simulink library "MBDyn_collision_activator"  (R2016b)
settings: Solver=VariableStepAuto  StartTime=0.0  StopTime=10.0  RelTol=1e-3
values from neighbouring files (symbols this model uses):
  coefficient_viscous_friction = 0.05    [multiple_points_platform_and_ball_characteristics.m]
  restitution_coefficient = 0.2    [multiple_points_platform_and_ball_characteristics.m]
undefined symbols (not defined in the file or in its folder): dz_at_rest, platform_damping_factor
undefined symbols (not defined in the file): Coulomb_friction_value, ctflag_threshold, delta_z_rest, dz_threshold, mu_z
libraries: simulink x4
settings Model: Creator=matteo  LastModifiedBy=matteo

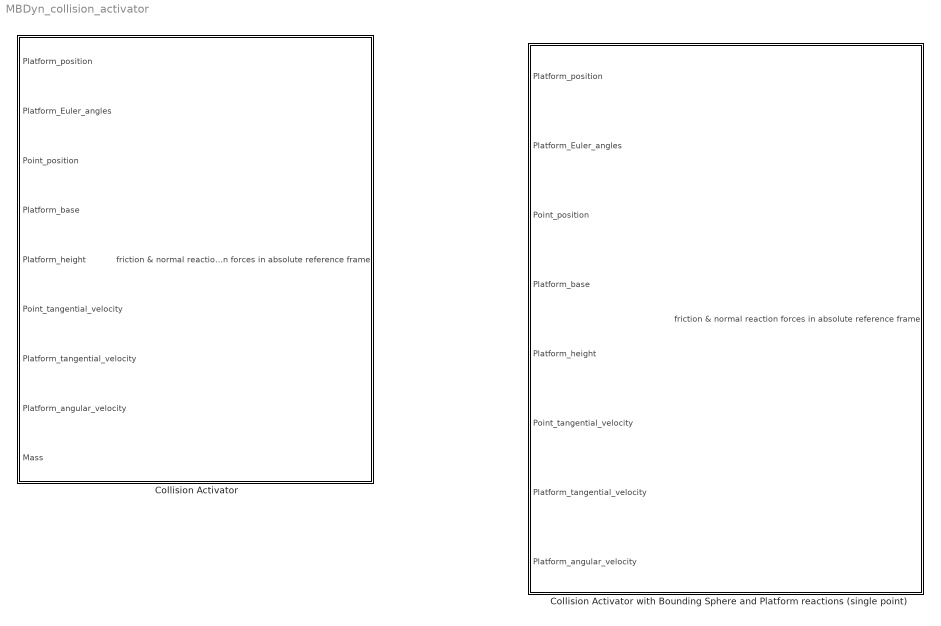
== system MBDyn_collision_activator ==
  Collision Activator : Subsystem  mask{coulomb_friction_value=Coulomb_friction_value, coefficient_viscous_friction=coefficient_viscous_friction, cosine_flag_threshold=ctflag_threshold, local_distance_from_gnd_threshold=dz_threshold, platform_damping_factor=mu_z, dz_at_rest=delta_z_rest}
      mask prompts: coulomb_friction_value "Coulomb friction value (offset)"; coefficient_viscous_friction "coefficient of viscous friction (gain)"; cosine_flag_threshold "cosine flag threshold"; local_distance_from_gnd_threshold "local distance from ground threshold"; platform_damping_factor "platform damping factor"; dz_at_rest "desired_platform deformation at rest"
      mask DialogControl MBDyn_collision_activator Prompt: MBDyn collision activator. Author: Matteo Daniele. This block models a simple point-to-rectangular platform collision interaction.
  Collision Activator with Bounding Sphere and Platform reactions (single point) : Subsystem  mask{mult_factor=10, coulomb_friction_value=0, coefficient_viscous_friction=0.05, cosine_flag_threshold=3.9, local_distance_from_gnd_threshold=0, ground_stiffness=1e9, restitution_coeff=0.8, impact_speed_threshold=0.2, reaction_force_exponential=3, force_sign=-1, dissipation_coefficient_model=Flores}
      mask prompts: mult_factor "bounding sphere platform multiplication factor"; coulomb_friction_value "Coulomb friction value (offset)"; coefficient_viscous_friction "coefficient of viscous friction (gain)"; cosine_flag_threshold "cosine flag threshold"; local_distance_from_gnd_threshold "local distance from ground threshold"; ground_stiffness "normal reaction stiffness"; restitution_coeff "restitution coefficient"; impact_speed_threshold "impact speed threshold"; reaction_force_exponential "reaction force exponential"; force_sign "reaction force sign (+1 or -1)"; dissipation_coefficient_model "dissipation coefficient model"
      mask TypeOptions dissipation_coefficient_model: Flores | Hunt Crossley | Lankarani Nikravesh
      mask DialogControl MBDyn_collision_activator Prompt: MBDyn collision activator. Author: Matteo Daniele. This block models a simple point-to-rectangular platform collision interaction.

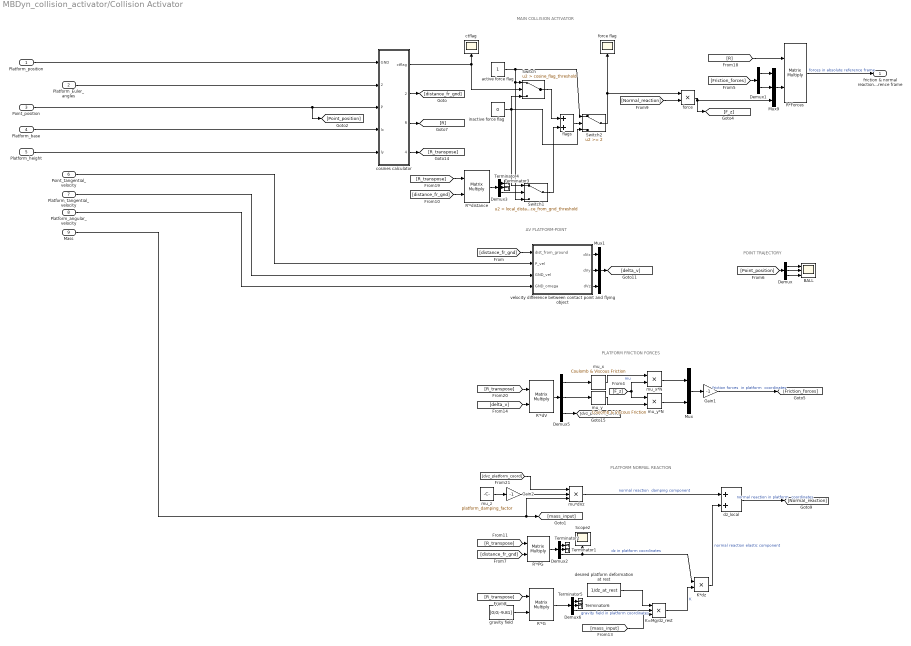
== system MBDyn_collision_activator/Collision Activator ==
  note: PLATFORM NORMAL REACTION
  note: PLATFORM FRICTION FORCES
  note: POINT TRAJECTORY
  note: ΔV PLATFORM-POINT
  note: MAIN COLLISION ACTIVATOR
  Platform_position : Inport
  Platform_Euler_angles : Inport  Port=2
  Point_position : Inport  Port=3
  Platform_base : Inport  Port=4
  Platform_height : Inport  Port=5
  Point_tangential_velocity : Inport  Port=6
  Platform_tangential_velocity : Inport  Port=7
  Platform_angular_velocity : Inport  Port=8
  Mass : Inport  Port=9
  BALL : Scope  NumInputPorts=3
  Demux{,2..3,5..6} (5 alike) : Demux  Outputs=3
  Demux1 : Demux  Outputs=2
  Gain1 : Gain  Gain=-1
  Gain2 : Gain  Gain=-1
  K*dz : Product
  K=Mg/dz_rest : Product  Inputs=3
  Mux : Mux  Inputs=2
  Mux1 : Mux  Inputs=3
  Mux9 : Mux  Inputs=3
  R'*G : Product  Multiplication=Matrix(*)
  R'*PG : Product  Multiplication=Matrix(*)
  R'*dV : Product  Multiplication=Matrix(*)
  R'*distance : Product  Multiplication=Matrix(*)
  R*Forces : Product  Multiplication=Matrix(*)
  Scope2 : Scope
  Switch : Switch  Criteria=u2 > Threshold  Threshold=cosine_flag_threshold
  Switch1 : Switch  Criteria=u2 > Threshold  Threshold=local_distance_from_gnd_threshold
  Switch2 : Switch  Threshold=2
  Terminator{1..6} (6 alike) : Terminator
  active force flag : Constant
  cosines calculator : MATLAB Function  TreatAsAtomicUnit=on
  ctflag : Scope
  desired platform deformation at rest : Constant  Value=1/dz_at_rest
  dz_local : Sum
  flags : Sum
  force : Product
  force flag : Scope
  gravity field : Constant  Value=[0;0;-9.81]
  inactive force flag : Constant  Value=0
  mu*dVz : Product  Inputs=3
  mu_x : simulink/Discontinuities/Coulomb & Viscous Friction  offset=coulomb_friction_value  gain=coefficient_viscous_friction
  mu_x*N : Product
  mu_y : simulink/Discontinuities/Coulomb & Viscous Friction  offset=coulomb_friction_value  gain=coefficient_viscous_friction
  mu_y*N : Product
  mu_z : Constant  Value=platform_damping_factor
  velocity difference between contact point and flying object : MATLAB Function  TreatAsAtomicUnit=on
  friction & normal reaction forces in absolute reference frame : Outport
  wires:
  active force flag/1 -> Switch/1, Switch1/3, Switch2/1
  dz_local/1 -> [Normal_reaction]  "normal reaction in platform  coordinates"
  Platform_height/1 -> cosines calculator/5(ly)
  cosines calculator/3(R) -> [R]
  cosines calculator/2(distance_PG) -> [distance_fr_gnd]
  [mass_input] -> K=Mg/dz_rest/3
  Demux6/3 -> K=Mg/dz_rest/2  "gravity field in platform coordinates"
  Platform_position/1 -> cosines calculator/1(GND)
  mu_y*N/1 -> Mux/2
  Demux5/3 -> [dvz_platform_coord]
  Demux2/2 -> Terminator1/1
  K=Mg/dz_rest/1 -> K*dz/2  "K"
  velocity difference between contact point and flying object/2(dVy) -> Mux1/2
  [distance_fr_gnd] -> R'*PG/2
  Demux/3 -> BALL/3
  [distance_fr_gnd] -> R'*distance/2
  Demux2/1 -> Terminator2/1
  Point_tangential_velocity/1 -> velocity difference between contact point and flying object/2(P_vel)
  Gain1/1 -> [Friction_forces]  "friction forces  in platform  coordinates"
  R*Forces/1 -> friction & normal reaction forces in absolute reference frame/1  "forces in absolute reference frame"
  Demux/1 -> BALL/1
  inactive force flag/1 -> Switch/3, Switch1/1, Switch2/3
  mu_x*N/1 -> Mux/1
  Platform_Euler_angles/1 -> cosines calculator/2(GND_Phi)
  Demux3/2 -> Terminator3/1
  mu*dVz/1 -> dz_local/1  "normal reaction  damping component"
  [F_z] -> mu_y*N/1, mu_x*N/2
  cosines calculator/1(ctflag) -> Switch/2, ctflag/1
  mu_y/1 -> mu_y*N/2
  Platform_tangential_velocity/1 -> velocity difference between contact point and flying object/3(GND_vel)
  Mux9/1 -> R*Forces/2
  velocity difference between contact point and flying object/1(dVx) -> Mux1/1
  [R_transpose] -> R'*G/1
  [R_transpose] -> R'*distance/1
  R'*dV/1 -> Demux5/1
  Point_position/1 -> cosines calculator/3(P), [Point_position]
  Gain2/1 -> mu*dVz/2
  R'*PG/1 -> Demux2/1
  Mass/1 -> mu*dVz/3, [mass_input]
  [Normal_reaction] -> force/2
  mu_x/1 -> mu_x*N/1  "mu"
  Mux1/1 -> [delta_v]
  [Point_position] -> Demux/1
  Switch2/1 -> force/1, force flag/1
  Demux1/2 -> Mux9/2
  Platform_angular_velocity/1 -> velocity difference between contact point and flying object/4(GND_omega)
  [R_transpose] -> R'*PG/1
  Demux6/1 -> Terminator5/1
  Demux3/3 -> Switch1/2
  Demux1/1 -> Mux9/1
  [R_transpose] -> R'*dV/1
  [Friction_forces] -> Demux1/1
  K*dz/1 -> dz_local/2  "normal reaction elastic component"
  Switch/1 -> flags/1
  force/1 -> [F_z], Mux9/3
  Demux/2 -> BALL/2
  Demux6/2 -> Terminator6/1
  flags/1 -> Switch2/2
  desired platform deformation at rest/1 -> K=Mg/dz_rest/1
  [distance_fr_gnd] -> velocity difference between contact point and flying object/1(dist_from_ground)
  Mux/1 -> Gain1/1
  mu_z/1 -> Gain2/1
  Demux3/1 -> Terminator4/1
  [dvz_platform_coord] -> mu*dVz/1
  cosines calculator/4(R_global_to_local) -> [R_transpose]
  Demux5/1 -> mu_x/1
  Demux5/2 -> mu_y/1
  velocity difference between contact point and flying object/3(dVz) -> Mux1/3
  R'*distance/1 -> Demux3/1
  R'*G/1 -> Demux6/1
  [R] -> R*Forces/1
  gravity field/1 -> R'*G/2
  [delta_v] -> R'*dV/2
  Switch1/1 -> flags/2
  Platform_base/1 -> cosines calculator/4(lx)
  Demux2/3 -> Scope2/1, K*dz/1  "dz in platform coordinates"

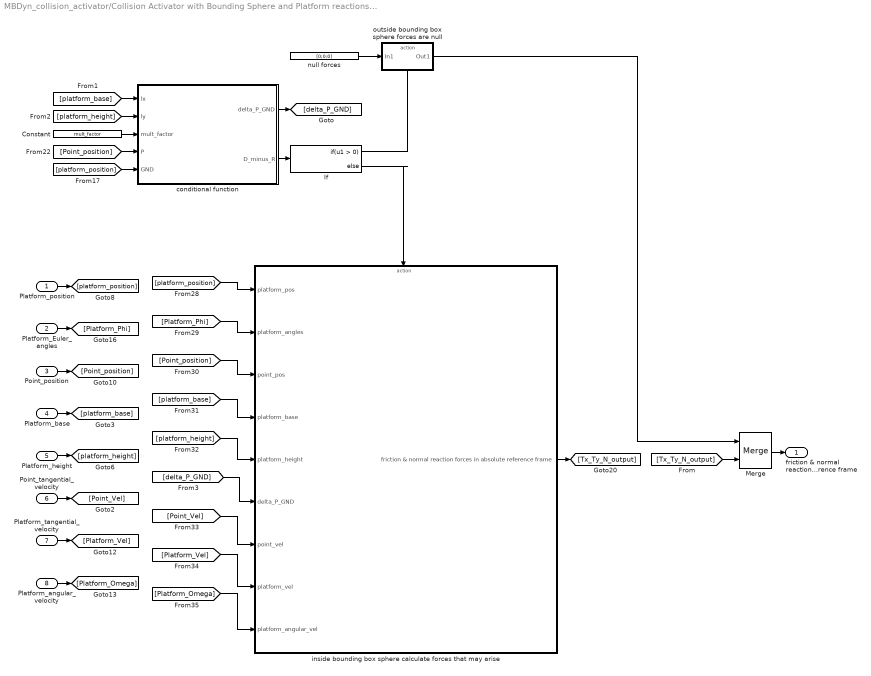
== system MBDyn_collision_activator/Collision Activator with Bounding Sphere and Platform reactions (single point) ==
  Platform_position : Inport
  Platform_Euler_angles : Inport  Port=2
  Point_position : Inport  Port=3
  Platform_base : Inport  Port=4
  Platform_height : Inport  Port=5
  Point_tangential_velocity : Inport  Port=6
  Platform_tangential_velocity : Inport  Port=7
  Platform_angular_velocity : Inport  Port=8
  Constant : Constant  Value=mult_factor
  If : If
  Merge : Merge
  conditional function : MATLAB Function  TreatAsAtomicUnit=on
  inside bounding box sphere calculate forces that may arise : Subsystem  TreatAsAtomicUnit=on
  null forces : Constant  Value=[0;0;0]
  outside bounding box sphere forces are null : Subsystem  TreatAsAtomicUnit=on
  friction & normal reaction forces in absolute reference frame : Outport
  wires:
  [delta_P_GND] -> inside bounding box sphere calculate forces that may arise/6(delta_P_GND)
  inside bounding box sphere calculate forces that may arise/1(friction & normal reaction forces in absolute reference frame) -> [Tx_Ty_N_output]
  null forces/1 -> outside bounding box sphere forces are null/1(In1)
  If/1 -> outside bounding box sphere forces are null/Action
  If/2 -> inside bounding box sphere calculate forces that may arise/Action
  [Platform_Omega] -> inside bounding box sphere calculate forces that may arise/9(platform_angular_vel)
  [Platform_Vel] -> inside bounding box sphere calculate forces that may arise/8(platform_vel)
  [Point_Vel] -> inside bounding box sphere calculate forces that may arise/7(point_vel)
  [platform_height] -> inside bounding box sphere calculate forces that may arise/5(platform_height)
  [platform_base] -> inside bounding box sphere calculate forces that may arise/4(platform_base)
  [Point_position] -> inside bounding box sphere calculate forces that may arise/3(point_pos)
  [Platform_Phi] -> inside bounding box sphere calculate forces that may arise/2(platform_angles)
  [platform_position] -> inside bounding box sphere calculate forces that may arise/1(platform_pos)
  conditional function/2(D_minus_R) -> If/1
  conditional function/1(delta_P_GND) -> [delta_P_GND]
  [Tx_Ty_N_output] -> Merge/2
  outside bounding box sphere forces are null/1(Out1) -> Merge/1
  Merge/1 -> friction & normal reaction forces in absolute reference frame/1
  Platform_Euler_angles/1 -> [Platform_Phi]
  Point_tangential_velocity/1 -> [Point_Vel]
  Platform_tangential_velocity/1 -> [Platform_Vel]
  Platform_angular_velocity/1 -> [Platform_Omega]
  [Point_position] -> conditional function/4(P)
  [platform_position] -> conditional function/5(GND)
  Constant/1 -> conditional function/3(mult_factor)
  Point_position/1 -> [Point_position]
  Platform_position/1 -> [platform_position]
  [platform_height] -> conditional function/2(ly)
  [platform_base] -> conditional function/1(lx)
  Platform_height/1 -> [platform_height]
  Platform_base/1 -> [platform_base]

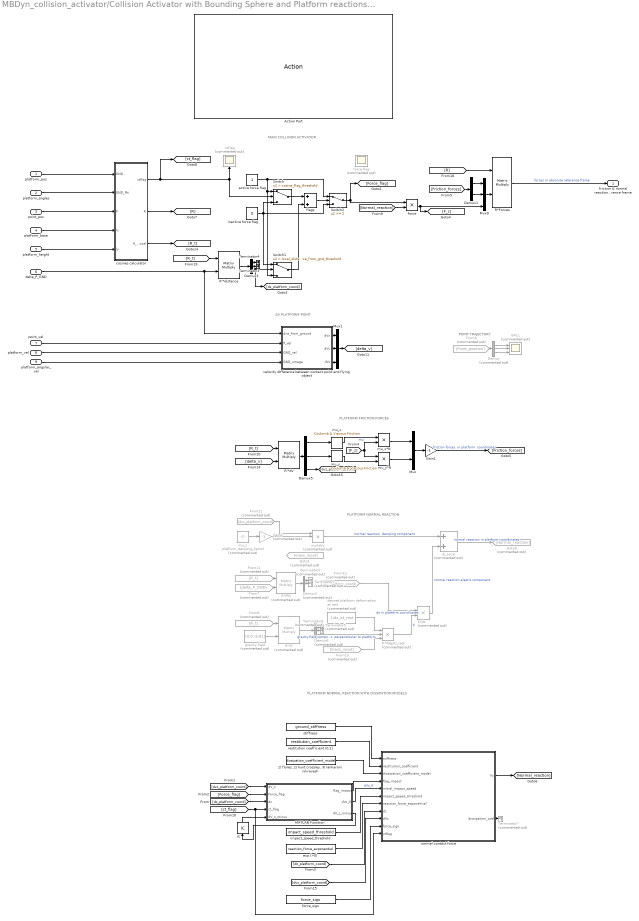
== system MBDyn_collision_activator/Collision Activator with Bounding Sphere and Platform reactions (single point)/inside bounding box sphere calculate forces that may arise ==
  note: PLATFORM NORMAL REACTION WITH DISSIPATION MODELS
  note: PLATFORM NORMAL REACTION
  note: PLATFORM FRICTION FORCES
  note: POINT TRAJECTORY
  note: ΔV PLATFORM-POINT
  note: MAIN COLLISION ACTIVATOR
  platform_pos : Inport
  platform_angles : Inport  Port=2
  point_pos : Inport  Port=3
  platform_base : Inport  Port=4
  platform_height : Inport  Port=5
  delta_P_GND : Inport  Port=6
  point_vel : Inport  Port=7
  platform_vel : Inport  Port=8
  platform_angular_vel : Inport  Port=9
  Action Port : ActionPort
  "1) flores, 2) hunt crossley, 3) lankarani nikravesh" : Constant  Value=dissipation_coefficient_model
  BALL : Scope  Commented=on  NumInputPorts=3
  Demux : Demux  Commented=on  Outputs=3
  Demux1 : Demux  Outputs=2
  Demux2 : Demux  Commented=on  Outputs=3
  Demux3 : Demux  Outputs=3
  Demux5 : Demux  Outputs=3
  Demux6 : Demux  Commented=on  Outputs=3
  From11 : From  Commented=on  GotoTag=R_t
  From12 : From  Commented=on  GotoTag=dz_platform_coord
  From13 : From  Commented=on  GotoTag=mass_input
  From21 : From  Commented=on  GotoTag=dvz_platform_coord
  From6 : From  Commented=on  GotoTag=Point_position
  From7 : From  Commented=on  GotoTag=delta_P_GND
  From8 : From  Commented=on  GotoTag=R_t
  Gain1 : Gain  Gain=-1
  Gain2 : Gain  Commented=on  Gain=-1
  Goto1 : Goto  Commented=on  GotoTag=mass_input
  Goto9 : Goto  Commented=on  GotoTag=Normal_reaction
  IC : InitialCondition  Value=0
  K*dz : Product  Commented=on
  K=Mg/dz_rest : Product  Commented=on  Inputs=3
  MATLAB Function : MATLAB Function  TreatAsAtomicUnit=on
  Mux : Mux  Inputs=2
  Mux1 : Mux  Inputs=3
  Mux9 : Mux  Inputs=3
  R'*G : Product  Commented=on  Multiplication=Matrix(*)
  R'*PG : Product  Commented=on  Multiplication=Matrix(*)
  R'*dV : Product  Multiplication=Matrix(*)
  R'*distance : Product  Multiplication=Matrix(*)
  R*Forces : Product  Multiplication=Matrix(*)
  Switch : Switch  Criteria=u2 > Threshold  Threshold=cosine_flag_threshold
  Switch1 : Switch  Criteria=u2 > Threshold  Threshold=local_distance_from_gnd_threshold
  Switch2 : Switch  Threshold=2
  Terminator{1..2,5..7} (5 alike) : Terminator  Commented=on
  Terminator3 : Terminator
  Terminator4 : Terminator
  active force flag : Constant
  cosines calculator : MATLAB Function  TreatAsAtomicUnit=on
  ctflag : Scope  Commented=on
  desired platform deformation at rest : Constant  Commented=on  Value=1/dz_at_rest
  dz_local : Sum  Commented=on
  exp (>0) : Constant  Value=reaction_force_exponential
  flags : Sum
  force : Product
  force flag : Scope  Commented=on
  force_sign : Constant  Value=force_sign
  gravity field : Constant  Commented=on  Value=[0;0;-9.81]
  impact_speed_threshold : Constant  Value=impact_speed_threshold
  inactive force flag : Constant  Value=0
  mu*dVz : Product  Commented=on  Inputs=3
  mu_x : simulink/Discontinuities/Coulomb & Viscous Friction  offset=coulomb_friction_value  gain=coefficient_viscous_friction
  mu_x*N : Product
  mu_y : simulink/Discontinuities/Coulomb & Viscous Friction  offset=coulomb_friction_value  gain=coefficient_viscous_friction
  mu_y*N : Product
  mu_z : Constant  Commented=on  Value=platform_damping_factor
  normal contact force : MATLAB Function  TreatAsAtomicUnit=on
  restitution coefficient (0,1] : Constant  Value=restitution_coefficient
  stiffness : Constant  Value=ground_stiffness
  velocity difference between contact point and flying object : MATLAB Function  TreatAsAtomicUnit=on
  friction & normal reaction forces in absolute reference frame : Outport
  wires:
  normal contact force/2(dissipation_coeff) -> Terminator7/1
  MATLAB Function/1(flag_impact) -> normal contact force/4(flag_impact)
  [Force_flag] -> MATLAB Function/2(Force_flag)
  [ct_flag] -> MATLAB Function/4(ct_flag), normal contact force/11(ctflag)
  [dz_platform_coord] -> MATLAB Function/3(dz)
  normal contact force/1(Fz) -> [Normal_reaction]
  MATLAB Function/3(dV_z_minus) -> IC/1
  force_sign/1 -> normal contact force/10(force_sign)
  [dvz_platform_coord] -> normal contact force/9(dVz)
  exp (>0)/1 -> normal contact force/7(reaction_force_exponential)
  impact_speed_threshold/1 -> normal contact force/6(impact_speed_threshold)
  "1) flores, 2) hunt crossley, 3) lankarani nikravesh"/1 -> normal contact force/3(dissipation_coefficient_model)
  restitution coefficient (0,1]/1 -> normal contact force/2(restitution_coefficient)
  stiffness/1 -> normal contact force/1(stiffness)
  IC/1 -> MATLAB Function/5("dV_z_minus ")
  [dz_platform_coord] -> normal contact force/8(dz)
  MATLAB Function/2(dVz_0) -> normal contact force/5(initial_impact_speed)  "dVz_0"
  [dvz_platform_coord] -> MATLAB Function/1(dV_z)
  platform_angular_vel/1 -> velocity difference between contact point and flying object/4(GND_omega)
  platform_vel/1 -> velocity difference between contact point and flying object/3(GND_vel)
  point_vel/1 -> velocity difference between contact point and flying object/2(P_vel)
  platform_height/1 -> cosines calculator/5(ly)
  platform_base/1 -> cosines calculator/4(lx)
  point_pos/1 -> cosines calculator/3(P)
  platform_angles/1 -> cosines calculator/2(GND_Phi)
  platform_pos/1 -> cosines calculator/1(GND)
  cosines calculator/2(R) -> [R]
  active force flag/1 -> Switch/1, Switch1/3, Switch2/1
  dz_local/1 -> Goto9/1  "normal reaction in platform  coordinates"
  From13/1 -> K=Mg/dz_rest/3
  Demux6/3 -> K=Mg/dz_rest/2  "gravity field component  perpendicular to platform"
  mu_y*N/1 -> Mux/2
  Demux5/3 -> [dvz_platform_coord]
  Demux2/2 -> Terminator1/1
  K=Mg/dz_rest/1 -> K*dz/2  "K"
  velocity difference between contact point and flying object/2(dVy) -> Mux1/2
  From7/1 -> R'*PG/2
  Demux/3 -> BALL/3
  Demux2/1 -> Terminator2/1
  Gain1/1 -> [Friction_forces]  "friction forces  in platform  coordinates"
  R*Forces/1 -> friction & normal reaction forces in absolute reference frame/1  "forces in absolute reference frame"
  Demux/1 -> BALL/1
  inactive force flag/1 -> Switch/3, Switch2/3, Switch1/1
  mu_x*N/1 -> Mux/1
  Demux3/2 -> Terminator3/1
  mu*dVz/1 -> dz_local/1  "normal reaction  damping component"
  [F_z] -> mu_y*N/1, mu_x*N/2
  cosines calculator/1(ctflag) -> Switch/2, ctflag/1, [ct_flag]
  mu_y/1 -> mu_y*N/2
  Mux9/1 -> R*Forces/2
  velocity difference between contact point and flying object/1(dVx) -> Mux1/1
  From8/1 -> R'*G/1
  [R_t] -> R'*distance/1
  R'*dV/1 -> Demux5/1
  Gain2/1 -> mu*dVz/2
  R'*PG/1 -> Demux2/1
  [Normal_reaction] -> force/2
  mu_x/1 -> mu_x*N/1  "mu"
  Mux1/1 -> [delta_v]
  From6/1 -> Demux/1
  Switch2/1 -> [Force_flag], force/1
  Demux1/2 -> Mux9/2
  From11/1 -> R'*PG/1
  Demux6/1 -> Terminator5/1
  Demux3/3 -> Switch1/2, [dz_platform_coord]
  Demux1/1 -> Mux9/1
  [R_t] -> R'*dV/1
  [Friction_forces] -> Demux1/1
  K*dz/1 -> dz_local/2  "normal reaction elastic component"
  Switch/1 -> flags/1
  force/1 -> [F_z], Mux9/3
  Demux/2 -> BALL/2
  Demux6/2 -> Terminator6/1
  flags/1 -> Switch2/2
  desired platform deformation at rest/1 -> K=Mg/dz_rest/1
  delta_P_GND/1 -> velocity difference between contact point and flying object/1(dist_from_ground), R'*distance/2
  Mux/1 -> Gain1/1
  mu_z/1 -> Gain2/1
  Demux3/1 -> Terminator4/1
  From21/1 -> mu*dVz/1
  cosines calculator/3(R_global_to_local) -> [R_t]
  Demux5/1 -> mu_x/1
  Demux5/2 -> mu_y/1
  velocity difference between contact point and flying object/3(dVz) -> Mux1/3
  R'*distance/1 -> Demux3/1
  R'*G/1 -> Demux6/1
  [R] -> R*Forces/1
  gravity field/1 -> R'*G/2
  [delta_v] -> R'*dV/2
  Switch1/1 -> flags/2
  From12/1 -> K*dz/1  "dz in platform coordinates"

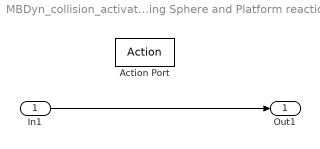
== system MBDyn_collision_activator/Collision Activator with Bounding Sphere and Platform reactions (single point)/outside bounding box sphere forces are null ==
  In1 : Inport
  Action Port : ActionPort
  Out1 : Outport
  wires:
  In1/1 -> Out1/1

== matlab function MBDyn_collision_activator/Collision Activator/cosines calculator ==
  data: GND input; ctflag output; GND_Phi input; P input; distance_PG output; lx input; ly input; R output; R_global_to_local output
function [ctflag,distance_PG,R,R_global_to_local] = fcn(GND,GND_Phi,P,lx,ly)
%% MATTEO DANIELE
% trying to create a contact constraint on platform that depends on the
% difference in position, speed, orientation and angular velocity between
% ground and "flying object"
n_vertices = 4;

% GND = [u(1);u(2);u(3)];
% GND_Phi = [u(4);u(5);u(6)];
% position of the point P ("flying object")
% P = [u(7);u(8);u(9)];

% rotation matrix to define all vertices
R = eul2rotm([GND_Phi(3) GND_Phi(2) GND_Phi(1)]);

% rotation matrix to define coordinates in the reference frame attached to
% the platfomr plane
R_global_to_local = R';
    
% initialization of z_normals and cosines
z_normals = zeros(3,n_vertices);
ct = zeros(1,n_vertices);
% initialization of distance vectors
PG = zeros(3,n_vertices);

% dimension of the platform along x 
% Length_x = u(10);
% dimension of the platform along y
% Length_y = u(11);

% rectangle of base Length_x and height Length_y
GND_vert = [ lx -lx -lx  lx
             ly  ly -ly -ly
              0  0   0   0  ];
               
for k = 1:n_vertices
    GND_vert(:,k) = GND + R*GND_vert(:,k);
%         distance vector between point and ground
        PG(:,k) = P-GND_vert(:,k);
%         normalization of the vector
        PG(:,k) = PG(:,k)/norm(PG(:,k));
end


% normals to planes
for k = 1:n_vertices-1
    z_normals(:,k) = cross(PG(:,k),PG(:,k+1));
    z_normals(:,k) = z_normals(:,k)/norm(z_normals(:,k));
end
z_normals(:,end) = cross(PG(:,end),PG(:,1));
z_normals(:,end) = z_normals(:,end)/norm(z_normals(:,end));

% platform plane normal (reference for cosine calculations)
z = cross(GND_vert(:,1)-GND,GND_vert(:,2)-GND);
z = z/norm(z);




% cosine of the angle between z and zij
for k = 1:n_vertices
    ct(k) = [z_normals(1,k) z_normals(2,k) z_normals(3,k)]*z;
end

% all cosines close to unit means that contact happens
ctflag = sum(ct);
% pass also the distance vector between "flying object" and ground
% reference point, it is useful to compute the arm for the angular speed of
% the velocity difference between point and platform
distance_PG = P-GND;

% ctflag close to 4 means that contact happens
% ideally when ctflag is 4 then contact happens, in reality ctflag must be
% over (or under) a certain limit to activate forces (eg: ctflag > 3.9)
% y(1,1) = ctflag;
% pass also the distance vector between "flying object" and ground
% reference point
% y(2:end,1) = P-GND;

== matlab function MBDyn_collision_activator/Collision Activator/velocity difference between contact point and flying object ==
  data: dist_from_ground input; dVx output; dVy output; P_vel input; GND_vel input; GND_omega input; dVz output
function [dVx,dVy,dVz] = fcn(dist_from_ground,P_vel,GND_vel,GND_omega)
%% MATTEO DANIELE
%  this function is intended to compute the relative velocity between the
%  contact point and the reference mass in order to model the surface
%  friction in a someway empirically

% distance between ground and "flying object" (for total speed)
% PG_distance = u(1:3);

% velocities useful to friction model
% P_vel = u(4:6);
% GND_vel = u(7:9);
% GND_omega = u(10:12);

% the contact point speed depends on the speed of GND node
V_Contact_Point = GND_vel + cross(GND_omega,dist_from_ground);

% speed difference between contact point and "flying object"
delta_V = P_vel-V_Contact_Point;

dVx = delta_V(1);
dVy = delta_V(2);
dVz = delta_V(3);

== matlab function MBDyn_collision_activator/Collision Activator with Bounding Sphere and Platform reactions (single point)/conditional function ==
  data: lx input; delta_P_GND output; ly input; mult_factor input; P input; GND input; D_minus_R output
function [delta_P_GND,D_minus_R] = fcn(lx,ly,mult_factor,P,GND)

% distance between point and platform center
delta_P_GND = P - GND;
% distance vector (norm of the distance)
delta_P_GND_norm = norm(delta_P_GND);

% bounding box sphere radius
% to be safe
if mult_factor <= 0
    mult_factor = 10;
end
bounding_sphere_radius = abs(mult_factor*max([lx ly]));

% difference between distance and bounding sphere radius
D_minus_R = delta_P_GND_norm - bounding_sphere_radius;

== matlab function MBDyn_collision_activator/Collision Activator with Bounding Sphere and Platform reactions (single point)/inside bounding box sphere calculate forces that may arise/MATLAB Function ==
  data: flag_impact output; dV_z input; Force_flag input; dz input; ct_flag input; dVz_0 output; dV_z_minus input; dV_z_minus output
function [flag_impact,dVz_0,dV_z_minus] = initial_impact_speed(dV_z,Force_flag,dz,ct_flag,dV_z_minus)
% dz: distance difference
% dVz: actual velocity difference
% dVz_minus: previous velocity difference
% dVz_0: initial impact speed
% no impact happens
% dVz_0 = 0;

    if dz > 0
        % if no compenetration then dVz_0 is not needed and dVz_minus updates
        % to the newest value of speed    
        dVz_0 = 0;
        dV_z_minus = dV_z;
        flag_impact = 0;
    else
       % impact happened
        flag_impact = 1;
       % active force flag: dVz_0 is the initial impact speed, and dVz_minus is
       % not updated anymore
        dVz_0 = dV_z_minus;
    end
    

end

== matlab function MBDyn_collision_activator/Collision Activator with Bounding Sphere and Platform reactions (single point)/inside bounding box sphere calculate forces that may arise/cosines calculator ==
  data: GND input; ctflag output; GND_Phi input; P input; lx input; ly input; R output; R_global_to_local output
function [ctflag,R,R_global_to_local] = fcn(GND,GND_Phi,P,lx,ly)
%% MATTEO DANIELE
% trying to create a contact constraint on platform that depends on the
% difference in position, speed, orientation and angular velocity between
% ground and "flying object"
n_vertices = 4;

% GND = [u(1);u(2);u(3)];
% GND_Phi = [u(4);u(5);u(6)];
% position of the point P ("flying object")
% P = [u(7);u(8);u(9)];

% rotation matrix to define all vertices
R = eul2rotm([GND_Phi(3) GND_Phi(2) GND_Phi(1)]);

% rotation matrix to define coordinates in the reference frame attached to
% the platfomr plane
R_global_to_local = R';
    
% initialization of z_normals and cosines
z_normals = zeros(3,n_vertices);
ct = zeros(1,n_vertices);
% initialization of distance vectors
PG = zeros(3,n_vertices);

% dimension of the platform along x 
% Length_x = u(10);
% dimension of the platform along y
% Length_y = u(11);

% rectangle of base Length_x and height Length_y
GND_vert = [ lx -lx -lx  lx
             ly  ly -ly -ly
              0  0   0   0  ];
               
for k = 1:n_vertices
    GND_vert(:,k) = GND + R*GND_vert(:,k);
%         distance vector between point and ground
        PG(:,k) = P-GND_vert(:,k);
%         normalization of the vector
        PG(:,k) = PG(:,k)/norm(PG(:,k));
end


% normals to planes
for k = 1:n_vertices-1
    z_normals(:,k) = cross(PG(:,k),PG(:,k+1));
    z_normals(:,k) = z_normals(:,k)/norm(z_normals(:,k));
end
z_normals(:,end) = cross(PG(:,end),PG(:,1));
z_normals(:,end) = z_normals(:,end)/norm(z_normals(:,end));

% platform plane normal (reference for cosine calculations)
z = cross(GND_vert(:,1)-GND,GND_vert(:,2)-GND);
z = z/norm(z);




% cosine of the angle between z and zij
for k = 1:n_vertices
    ct(k) = [z_normals(1,k) z_normals(2,k) z_normals(3,k)]*z;
end

% all cosines close to unit means that contact happens
ctflag = sum(ct);
% distance from ground is computed at the beginning to trigger the
% activator
% distance_PG = P-GND;

% ctflag close to 4 means that contact happens
% ideally when ctflag is 4 then contact happens, in reality ctflag must be
% over (or under) a certain limit to activate forces (eg: ctflag > 3.9)
% y(1,1) = ctflag;
% pass also the distance vector between "flying object" and ground
% reference point
% y(2:end,1) = P-GND;

== matlab function MBDyn_collision_activator/Collision Activator with Bounding Sphere and Platform reactions (single point)/inside bounding box sphere calculate forces that may arise/normal contact force ==
  data: stiffness input; Fz output; restitution_coefficient input; dissipation_coefficient_model input; flag_impact input; dissipation_coeff output; initial_impact_speed input; impact_speed_threshold input; reaction_force_exponential input; dz input; dVz input; force_sign input; ctflag input
function [Fz,dissipation_coeff] = normal_contact_force(stiffness,...
                                        restitution_coefficient,...
                                        dissipation_coefficient_model,...
                                        flag_impact,...
                                        initial_impact_speed,...
                                        impact_speed_threshold,...
                                        reaction_force_exponential,...
                                        dz,...
                                        dVz,...
                                        force_sign,...
                                        ctflag)

dissipation_coeff = 0;
% dissipation coefficient calculator
if flag_impact < 1
    Fz = 0;
    dissipation_coeff = 0;

else
    
    if abs(initial_impact_speed) < impact_speed_threshold

        dissipation_coeff = 0;

    else

        % flores
        if dissipation_coefficient_model == 1

            dissipation_coeff = (8/5)*stiffness*(1-restitution_coefficient)/(restitution_coefficient*initial_impact_speed);

        % hunt crossley
        elseif dissipation_coefficient_model == 2

            dissipation_coeff = (3/2)*stiffness*(1-restitution_coefficient)/initial_impact_speed;

        % lankarani nikravesh
        elseif dissipation_coefficient_model == 3

            dissipation_coeff = (3/4)*stiffness*(1-restitution_coefficient^2)/initial_impact_speed;

        end

    end

    % computation of the normal contact force
    Fz = force_sign*(dz^(reaction_force_exponential))*(stiffness + dissipation_coeff*dVz);

end

% saturation: if out of platform (ctflag = 0) then force is reset
Fz = Fz*ctflag;

== matlab function MBDyn_collision_activator/Collision Activator with Bounding Sphere and Platform reactions (single point)/inside bounding box sphere calculate forces that may arise/velocity difference between contact point and flying object ==
  data: dist_from_ground input; dVx output; dVy output; P_vel input; GND_vel input; GND_omega input; dVz output
function [dVx,dVy,dVz] = fcn(dist_from_ground,P_vel,GND_vel,GND_omega)
%% MATTEO DANIELE
%  this function is intended to compute the relative velocity between the
%  contact point and the reference mass in order to model the surface
%  friction in a someway empirically

% distance between ground and "flying object" (for total speed)
% PG_distance = u(1:3);

% velocities useful to friction model
% P_vel = u(4:6);
% GND_vel = u(7:9);
% GND_omega = u(10:12);

% the contact point speed depends on the speed of GND node
V_Contact_Point = GND_vel + cross(GND_omega,dist_from_ground);

% speed difference between contact point and "flying object"
delta_V = P_vel-V_Contact_Point;

dVx = delta_V(1);
dVy = delta_V(2);
dVz = delta_V(3);
